simulink model "Heading_Guide_110"  (Simulink 8.7)
settings: Solver=ode45  StartTime=0.0  StopTime=10.0  RelTol=1e-3
undefined symbols (not defined in the file or in its folder): DiscIntNeverNeededParam
libraries: simulink x1, discretizing x1
settings Model: Creator=arnaud  LastModifiedBy=bourbouh
settings DataIOCC: SignalLoggingSaveFormat=ModelDataLogs
settings OptimizationCC: ExpressionDepthLimit=2147483647
settings DebuggingCC: SolverPrmCheckMsg=warning  FcnCallInpInsideContextMsg=UseLocalSettings  StateNameClashWarn=warning  StrictBusMsg=Warning
settings GRTTargetCC: GeneratePreprocessorConditionals=Use local settings  CombineOutputUpdateFcns=off  GRTInterface=on

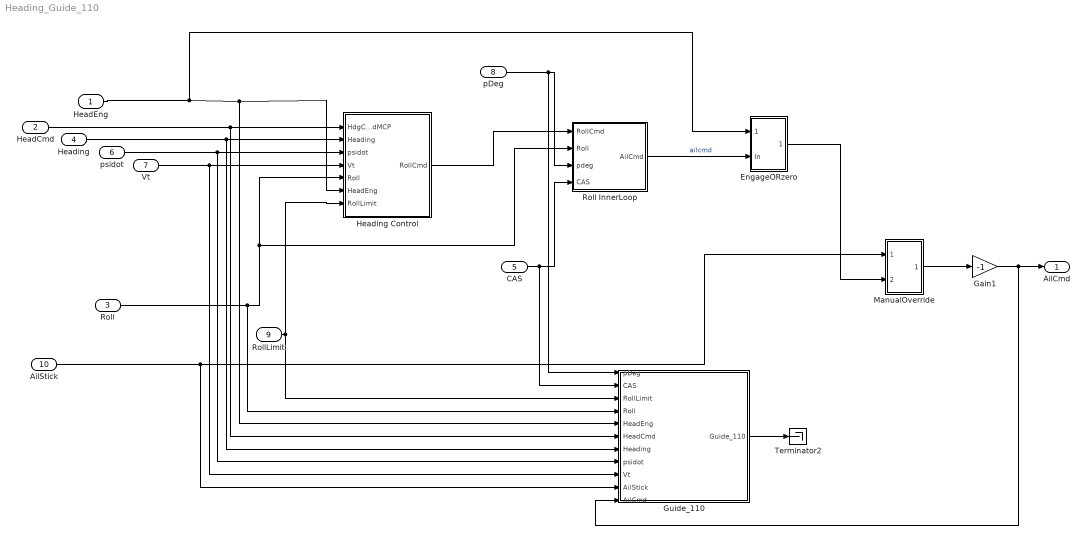
== system Heading_Guide_110 ==
  HeadEng : Inport  OutDataTypeStr=boolean
  HeadCmd : Inport  Port=2  OutDataTypeStr=double
  Roll : Inport  Port=3  OutDataTypeStr=double
  Heading : Inport  Port=4  OutDataTypeStr=double
  CAS : Inport  Port=5  OutDataTypeStr=double
  psidot : Inport  Port=6  OutDataTypeStr=double
  Vt : Inport  Port=7  OutDataTypeStr=double
  pDeg : Inport  Port=8  OutDataTypeStr=double
  RollLimit : Inport  Port=9  OutDataTypeStr=double
  AilStick : Inport  Port=10  OutDataTypeStr=double
  EngageORzero : Subsystem
  Gain1 : Gain  RequirementInfo={} %GIDa_2f421c02_996e_46c9_ac2a_3c25b016b229  Gain=-1  SaturateOnIntegerOverflow=on  OutDataTypeStr=Inherit: Same as input  ParamDataTypeStr=Inherit: Same as input
  Guide_110 : Subsystem  TreatAsAtomicUnit=on  mask(Observer){AnnotationType=ensures, ObserverType=ellipsoid}
      mask prompts: AnnotationType "Type of annotation (pre/post...)"; ObserverType "Observer type"
      mask help:
      | Set an observer for the system.
      | The annotation type parameter sets the type of observer:
      | - requires : pre-condition
      | - ensures : post-condition
      | - assert : an assertion
      | - observer : the observer computes a special type of properties
      mask TypeOptions AnnotationType: ensures | requires | assert | observer
      mask Callback AnnotationType:
      | paramStr = get_param(gcb, 'MaskValues');
      | 
      | if strcmp(paramStr{1}(1),'o')
      |     set_param(gcb,'MaskVisibilities',{'on';'on'});
      |     paramStr{2} = 'ellipsoid';
      |     set_param(gcb,'MaskValues',paramStr);
      | else
      |     set_param(gcb,'MaskVisibilities',{'on';'off'});
      | end
      mask Callback ObserverType:
      | paramStr = get_param(gcb, 'MaskValues');
      | 
      | if strcmp(paramStr{1}(1),'observer')
      |     set_param(gcb,'MaskVisibilities',{'on';'on'});
      |     paramStr{2} = 'ellipsoid';
      |     set_param(gcb,'MaskValues',paramStr);
      | else
      |     set_param(gcb,'MaskVisibilities',{'on';'off'});
      | end
      mask Display:
      | color('red');
      | text(0.5, 0.5, 'Observer Block', 'horizontalAlignment', 'center');
  Heading Control : Subsystem  RequirementInfo={'other' '..\..\tcm_requirements.docx' '@Simulink_requirement_item_16' 'true' 'Heading Control' '' }  TreatAsAtomicUnit=on
  ManualOverride : Subsystem
  Roll InnerLoop : Subsystem  RequirementInfo={'other' '..\..\tcm_requirements.docx' '@Simulink_requirement_item_18' 'true' 'Roll InnerLoop' '' }  TreatAsAtomicUnit=on
  Terminator2 : Terminator
  AilCmd : Outport
  wires:
  pDeg/1 -> Roll InnerLoop/3(pdeg), Guide_110/1(pDeg)
  Vt/1 -> Heading Control/4(Vt), Guide_110/9(Vt)
  psidot/1 -> Heading Control/3(psidot), Guide_110/8(psidot)
  Heading/1 -> Heading Control/2(Heading), Guide_110/7(Heading)
  Roll/1 -> Heading Control/5(Roll), Roll InnerLoop/2(Roll), Guide_110/4(Roll)
  Heading Control/1(RollCmd) -> Roll InnerLoop/1(RollCmd)
  Roll InnerLoop/1(AilCmd) -> EngageORzero/2(In)  "ailcmd"
  HeadEng/1 -> EngageORzero/1(Engage), Heading Control/6(HeadEng), Guide_110/5(HeadEng)
  CAS/1 -> Roll InnerLoop/4(CAS), Guide_110/2(CAS)
  RollLimit/1 -> Heading Control/7(RollLimit), Guide_110/3(RollLimit)
  ManualOverride/1(Out) -> Gain1/1
  AilStick/1 -> ManualOverride/1(Man), Guide_110/10(AilStick)
  Gain1/1 -> AilCmd/1, Guide_110/11(AilCmd)
  EngageORzero/1(Out) -> ManualOverride/2(Auto)
  HeadCmd/1 -> Heading Control/1(HdgCmdMCP), Guide_110/6(HeadCmd)
  Guide_110/1(Guide_110) -> Terminator2/1

== system Heading_Guide_110/EngageORzero ==
  Engage : Inport
  In : Inport  Port=2
  Logical Operator5 : Logic  RequirementInfo={} %GIDa_7add67f6_200e_4459_8afc_a50a3802c341  AllPortsSameDT=off  OutDataTypeStr=boolean
  Switch1 : Switch  RequirementInfo={} %GIDa_a1777089_6daf_41d2_9e69_9356c4782e25  Threshold=0.5
  zero10 : Constant  RequirementInfo={} %GIDa_d889400f_b153_4cfc_a180_15b84145f1e0
  zero9 : Constant  RequirementInfo={} %GIDa_9027fd24_3b48_4acd_a774_517fb1aa3516  Value=0
  Out : Outport
  wires:
  Engage/1 -> Logical Operator5/1
  zero10/1 -> Logical Operator5/2
  zero9/1 -> Switch1/3
  In/1 -> Switch1/1
  Logical Operator5/1 -> Switch1/2
  Switch1/1 -> Out/1

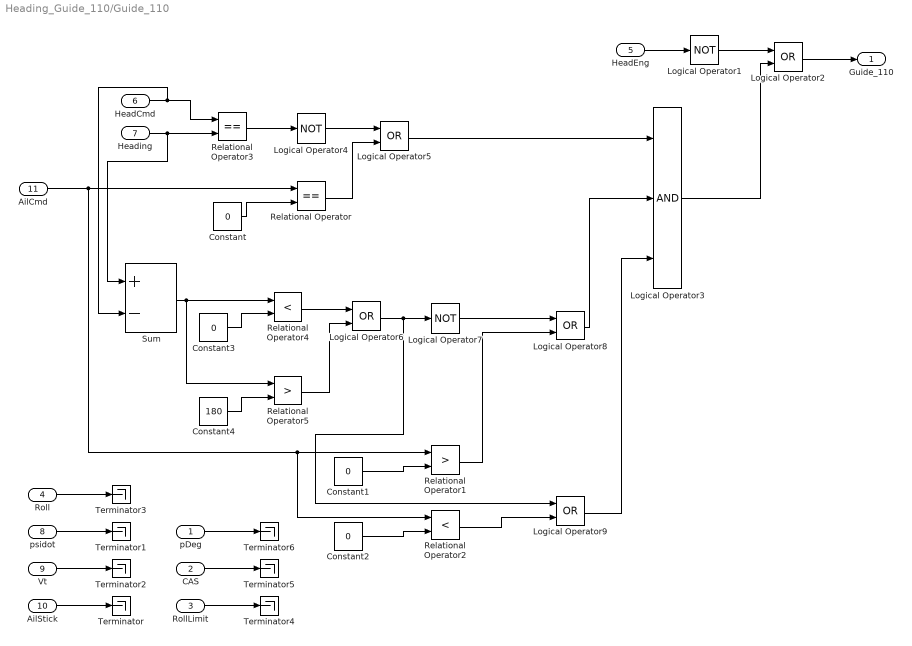
== system Heading_Guide_110/Guide_110 ==
  pDeg : Inport
  CAS : Inport  Port=2
  RollLimit : Inport  Port=3
  Roll : Inport  Port=4
  HeadEng : Inport  Port=5
  HeadCmd : Inport  Port=6
  Heading : Inport  Port=7
  psidot : Inport  Port=8
  Vt : Inport  Port=9
  AilStick : Inport  Port=10
  AilCmd : Inport  Port=11
  Constant{,1..3} (4 alike) : Constant  Value=0
  Constant4 : Constant  Value=180
  Logical Operator1 : Logic  Operator=NOT  AllPortsSameDT=off  OutDataTypeStr=boolean
  Logical Operator{2,5..6,8..9} (5 alike) : Logic  Operator=OR  AllPortsSameDT=off  OutDataTypeStr=boolean
  Logical Operator3 : Logic  Inputs=3  AllPortsSameDT=off  OutDataTypeStr=boolean
  Logical Operator4 : Logic  Operator=NOT  AllPortsSameDT=off  OutDataTypeStr=boolean
  Logical Operator7 : Logic  Operator=NOT  AllPortsSameDT=off  OutDataTypeStr=boolean
  Relational Operator : RelationalOperator  Operator===  OutDataTypeStr=boolean
  Relational Operator1 : RelationalOperator  Operator=>  OutDataTypeStr=boolean
  Relational Operator2 : RelationalOperator  Operator=<  OutDataTypeStr=boolean
  Relational Operator3 : RelationalOperator  Operator===  OutDataTypeStr=boolean
  Relational Operator4 : RelationalOperator  Operator=<  OutDataTypeStr=boolean
  Relational Operator5 : RelationalOperator  Operator=>  OutDataTypeStr=boolean
  Sum : Sum  Inputs=+-
  Terminator{,1..6} (7 alike) : Terminator
  Guide_110 : Outport
  wires:
  AilStick/1 -> Terminator/1
  Vt/1 -> Terminator2/1
  psidot/1 -> Terminator1/1
  Roll/1 -> Terminator3/1
  RollLimit/1 -> Terminator4/1
  CAS/1 -> Terminator5/1
  pDeg/1 -> Terminator6/1
  HeadEng/1 -> Logical Operator1/1
  Logical Operator1/1 -> Logical Operator2/1
  Logical Operator2/1 -> Guide_110/1
  AilCmd/1 -> Relational Operator/1, Relational Operator1/1, Relational Operator2/1
  Constant/1 -> Relational Operator/2
  Constant1/1 -> Relational Operator1/2
  Constant2/1 -> Relational Operator2/2
  Logical Operator4/1 -> Logical Operator5/1
  Relational Operator3/1 -> Logical Operator4/1
  Relational Operator/1 -> Logical Operator5/2
  Logical Operator5/1 -> Logical Operator3/1
  Sum/1 -> Relational Operator4/1, Relational Operator5/1
  Constant3/1 -> Relational Operator4/2
  Relational Operator4/1 -> Logical Operator6/1
  Constant4/1 -> Relational Operator5/2
  Relational Operator5/1 -> Logical Operator6/2
  HeadCmd/1 -> Relational Operator3/1, Sum/2
  Heading/1 -> Relational Operator3/2, Sum/1
  Logical Operator6/1 -> Logical Operator7/1, Logical Operator9/1
  Logical Operator7/1 -> Logical Operator8/1
  Relational Operator1/1 -> Logical Operator8/2
  Logical Operator8/1 -> Logical Operator3/2
  Relational Operator2/1 -> Logical Operator9/2
  Logical Operator9/1 -> Logical Operator3/3
  Logical Operator3/1 -> Logical Operator2/2

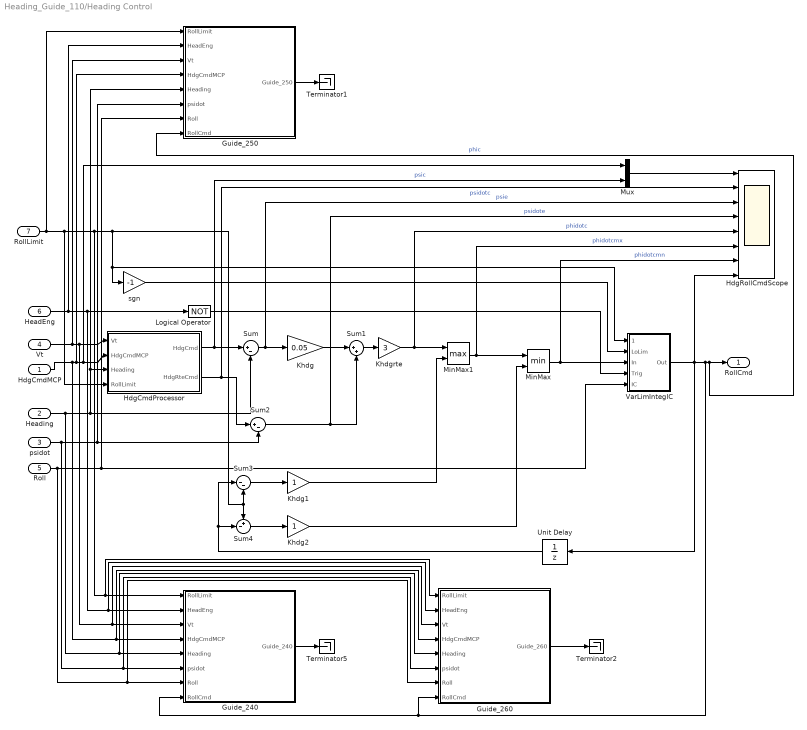
== system Heading_Guide_110/Heading Control ==
  HdgCmdMCP : Inport  RequirementInfo={} %GIDa_afcd05d1_a9dc_45a7_a8f8_7136ccc61726
  Heading : Inport  RequirementInfo={} %GIDa_19b80fe4_d265_482c_b709_18db80a7cdf3  Port=2
  psidot : Inport  RequirementInfo={} %GIDa_e421e82d_0cc7_4ad7_ac7a_9fb430d189d5  Port=3
  Vt : Inport  RequirementInfo={} %GIDa_9daf3e20_e00e_4f36_b534_d9747a241338  Port=4
  Roll : Inport  RequirementInfo={} %GIDa_8629ba77_a751_4097_af53_617eaa1017be  Port=5
  HeadEng : Inport  RequirementInfo={} %GIDa_dadb1310_2bf4_48cf_8970_85174d784ee3  Port=6
  RollLimit : Inport  Port=7
  Guide_240 : Subsystem  TreatAsAtomicUnit=on  mask(Observer){AnnotationType=ensures, ObserverType=ellipsoid}
      mask prompts: AnnotationType "Type of annotation (pre/post...)"; ObserverType "Observer type"
      mask help:
      | Set an observer for the system.
      | The annotation type parameter sets the type of observer:
      | - requires : pre-condition
      | - ensures : post-condition
      | - assert : an assertion
      | - observer : the observer computes a special type of properties
      mask TypeOptions AnnotationType: ensures | requires | assert | observer
      mask Callback AnnotationType:
      | paramStr = get_param(gcb, 'MaskValues');
      | 
      | if strcmp(paramStr{1}(1),'o')
      |     set_param(gcb,'MaskVisibilities',{'on';'on'});
      |     paramStr{2} = 'ellipsoid';
      |     set_param(gcb,'MaskValues',paramStr);
      | else
      |     set_param(gcb,'MaskVisibilities',{'on';'off'});
      | end
      mask Callback ObserverType:
      | paramStr = get_param(gcb, 'MaskValues');
      | 
      | if strcmp(paramStr{1}(1),'observer')
      |     set_param(gcb,'MaskVisibilities',{'on';'on'});
      |     paramStr{2} = 'ellipsoid';
      |     set_param(gcb,'MaskValues',paramStr);
      | else
      |     set_param(gcb,'MaskVisibilities',{'on';'off'});
      | end
      mask Display:
      | color('red');
      | text(0.5, 0.5, 'Observer Block', 'horizontalAlignment', 'center');
  Guide_250 : Subsystem  TreatAsAtomicUnit=on  mask(Observer){AnnotationType=ensures, ObserverType=ellipsoid}
      mask prompts: AnnotationType "Type of annotation (pre/post...)"; ObserverType "Observer type"
      mask help:
      | Set an observer for the system.
      | The annotation type parameter sets the type of observer:
      | - requires : pre-condition
      | - ensures : post-condition
      | - assert : an assertion
      | - observer : the observer computes a special type of properties
      mask TypeOptions AnnotationType: ensures | requires | assert | observer
      mask Callback AnnotationType:
      | paramStr = get_param(gcb, 'MaskValues');
      | 
      | if strcmp(paramStr{1}(1),'o')
      |     set_param(gcb,'MaskVisibilities',{'on';'on'});
      |     paramStr{2} = 'ellipsoid';
      |     set_param(gcb,'MaskValues',paramStr);
      | else
      |     set_param(gcb,'MaskVisibilities',{'on';'off'});
      | end
      mask Callback ObserverType:
      | paramStr = get_param(gcb, 'MaskValues');
      | 
      | if strcmp(paramStr{1}(1),'observer')
      |     set_param(gcb,'MaskVisibilities',{'on';'on'});
      |     paramStr{2} = 'ellipsoid';
      |     set_param(gcb,'MaskValues',paramStr);
      | else
      |     set_param(gcb,'MaskVisibilities',{'on';'off'});
      | end
      mask Display:
      | color('red');
      | text(0.5, 0.5, 'Observer Block', 'horizontalAlignment', 'center');
  Guide_260 : Subsystem  TreatAsAtomicUnit=on  mask(Observer){AnnotationType=ensures, ObserverType=ellipsoid}
      mask prompts: AnnotationType "Type of annotation (pre/post...)"; ObserverType "Observer type"
      mask help:
      | Set an observer for the system.
      | The annotation type parameter sets the type of observer:
      | - requires : pre-condition
      | - ensures : post-condition
      | - assert : an assertion
      | - observer : the observer computes a special type of properties
      mask TypeOptions AnnotationType: ensures | requires | assert | observer
      mask Callback AnnotationType:
      | paramStr = get_param(gcb, 'MaskValues');
      | 
      | if strcmp(paramStr{1}(1),'o')
      |     set_param(gcb,'MaskVisibilities',{'on';'on'});
      |     paramStr{2} = 'ellipsoid';
      |     set_param(gcb,'MaskValues',paramStr);
      | else
      |     set_param(gcb,'MaskVisibilities',{'on';'off'});
      | end
      mask Callback ObserverType:
      | paramStr = get_param(gcb, 'MaskValues');
      | 
      | if strcmp(paramStr{1}(1),'observer')
      |     set_param(gcb,'MaskVisibilities',{'on';'on'});
      |     paramStr{2} = 'ellipsoid';
      |     set_param(gcb,'MaskValues',paramStr);
      | else
      |     set_param(gcb,'MaskVisibilities',{'on';'off'});
      | end
      mask Display:
      | color('red');
      | text(0.5, 0.5, 'Observer Block', 'horizontalAlignment', 'center');
  HdgCmdProcessor : Subsystem  RequirementInfo={} %GIDa_3cb77e5f_f630_4f22_88a8_7528bfceb83f
  HdgRollCmdScope : Scope  NumInputPorts=8
      settings: RequirementInfo={} %GIDa_5fbe2135_fdf1_4f64_a179_faa1710ae21e
  Khdg : Gain  RequirementInfo={} %GIDa_abf81b08_c210_4343_b4da_5a7e229caeb6  Gain=0.05
  Khdg1 : Gain  RequirementInfo={} %GIDa_7a7a35ca_24a5_4d20_bc30_55deea16462c
  Khdg2 : Gain  RequirementInfo={} %GIDa_57191899_7ee5_4454_897a_7009651ed5fb
  Khdgrte : Gain  RequirementInfo={} %GIDa_bcc6a420_18f3_43f0_aaa1_aaa1bbf90f64  Gain=3
  Logical Operator : Logic  RequirementInfo={} %GIDa_5ad405ac_0a88_4b96_aa0e_75483351ee25  Operator=NOT  AllPortsSameDT=off  OutDataTypeStr=boolean
  MinMax : MinMax  RequirementInfo={} %GIDa_4b9381d8_eb85_418b_a975_85846d5ca8c2  Inputs=2
  MinMax1 : MinMax  RequirementInfo={} %GIDa_b40e082d_0fb2_4088_baf4_e9a71be9bcc1  Function=max  Inputs=2
  Mux : Mux  RequirementInfo={} %GIDa_0e83f6c6_ae04_43dd_95fe_a79ec32b40e2  Inputs=2
  Sum : Sum  RequirementInfo={} %GIDa_b89885fc_f86c_4a50_8ce5_47d0488bdc1c  Inputs=|+-
  Sum1 : Sum  RequirementInfo={} %GIDa_40ec6862_b1f8_4f97_ae14_1eadabbceb30  Inputs=|++
  Sum2 : Sum  RequirementInfo={} %GIDa_307d6880_3ab8_4deb_90e0_d68f11d87c85  Inputs=|+-
  Sum3 : Sum  RequirementInfo={} %GIDa_ebb8b765_7f4a_435f_be61_680d3199141b  Inputs=|--
  Sum4 : Sum  RequirementInfo={} %GIDa_05638559_562a_476e_9e4c_91124434a43b  Inputs=+-|
  Terminator1 : Terminator
  Terminator2 : Terminator
  Terminator5 : Terminator
  Unit Delay : UnitDelay  SampleTime=-1
  VarLimIntegIC : Subsystem  RequirementInfo={} %GIDa_7da7eaf5_9731_498e_9aad_b41279918004
  sgn : Gain  RequirementInfo={} %GIDa_84e2dc00_f2e5_41f4_89ce_c9fef234974f  Gain=-1
  RollCmd : Outport  RequirementInfo={} %GIDa_aa862f7f_5d4e_408f_b8c4_26b4ce96fbda
  wires:
  Heading/1 -> Guide_250/5(Heading), HdgCmdProcessor/3(Heading), Sum/2, Guide_240/5(Heading), Guide_260/5(Heading)
  HdgCmdProcessor/1(HdgCmd) -> Sum/1, Mux/2  "psic"
  Sum/1 -> Khdg/1, HdgRollCmdScope/3  "psie"
  Khdg/1 -> Sum1/1
  Sum2/1 -> Sum1/2, HdgRollCmdScope/4  "psidote"
  HdgCmdProcessor/2(HdgRteCmd) -> Sum2/1, HdgRollCmdScope/2  "psidotc"
  psidot/1 -> Sum2/2, Guide_250/6(psidot), Guide_240/6(psidot), Guide_260/6(psidot)
  Vt/1 -> HdgCmdProcessor/1(Vt), Guide_240/3(Vt), Guide_260/3(Vt), Guide_250/3(Vt)
  HdgCmdMCP/1 -> HdgCmdProcessor/2(HdgCmdMCP), Mux/1, Guide_250/4(HdgCmdMCP), Guide_240/4(HdgCmdMCP), Guide_260/4(HdgCmdMCP)
  VarLimIntegIC/1(Out) -> Unit Delay/1, HdgRollCmdScope/8, RollCmd/1, Guide_250/8(RollCmd), Guide_240/8(RollCmd), Guide_260/8(RollCmd)  "phic"
  RollLimit/1 -> Sum4/1, Sum3/2, VarLimIntegIC/1(UpLim), sgn/1, Guide_240/1(RollLimit), Guide_260/1(RollLimit), HdgCmdProcessor/4(RollLimit), Guide_250/1(RollLimit)
  sgn/1 -> VarLimIntegIC/2(LoLim)
  Sum1/1 -> Khdgrte/1
  MinMax1/1 -> MinMax/1, HdgRollCmdScope/6  "phidotcmx"
  MinMax/1 -> VarLimIntegIC/3(In), HdgRollCmdScope/7  "phidotcmn"
  HeadEng/1 -> Logical Operator/1, Guide_240/2(HeadEng), Guide_260/2(HeadEng), Guide_250/2(HeadEng)
  Sum3/1 -> Khdg1/1
  Sum4/1 -> Khdg2/1
  Khdg1/1 -> MinMax1/2
  Khdg2/1 -> MinMax/2
  Roll/1 -> VarLimIntegIC/5(IC), Guide_250/7(Roll), Guide_240/7(Roll), Guide_260/7(Roll)
  Khdgrte/1 -> MinMax1/1, HdgRollCmdScope/5  "phidotc"
  Logical Operator/1 -> VarLimIntegIC/4(Trig)
  Mux/1 -> HdgRollCmdScope/1
  Guide_240/1(Guide_240) -> Terminator5/1
  Guide_250/1(Guide_250) -> Terminator1/1
  Guide_260/1(Guide_260) -> Terminator2/1
  Unit Delay/1 -> Sum3/1, Sum4/2

== system Heading_Guide_110/ManualOverride ==
  Man : Inport
  Auto : Inport  Port=2
  Switch1 : Switch  RequirementInfo={} %GIDa_5800ea93_45af_42da_974c_4cd975d0b8c8  Criteria=u2 ~= 0  Threshold=0.5
  Out : Outport
  wires:
  Man/1 -> Switch1/3, Switch1/2
  Auto/1 -> Switch1/1
  Switch1/1 -> Out/1

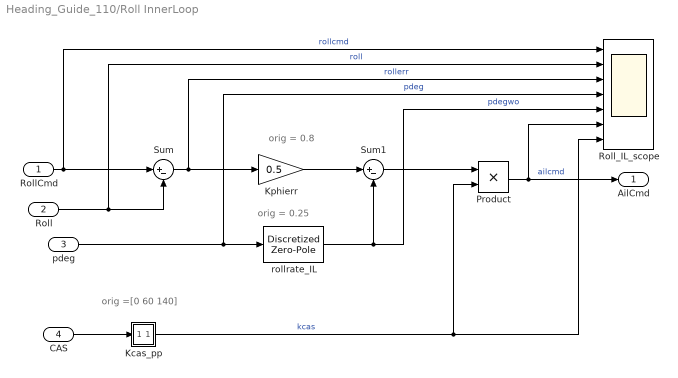
== system Heading_Guide_110/Roll InnerLoop ==
  note: orig =[0 60 140]
  note: orig = 0.25
  note: orig = 0.8
  RollCmd : Inport  RequirementInfo={} %GIDa_549f9d91_ca5c_4ec7_bf56_cf05f3793396
  Roll : Inport  RequirementInfo={} %GIDa_d885705c_af8c_4e18_b4d1_2f073687ea2c  Port=2
  pdeg : Inport  RequirementInfo={} %GIDa_ba7aa095_15b8_4f85_9051_8b947d28a24d  Port=3
  CAS : Inport  RequirementInfo={} %GIDa_defe4f55_1722_479a_b684_dc07a497c4ef  Port=4
  Kcas_pp : Subsystem  TreatAsAtomicUnit=on
  Kphierr : Gain  RequirementInfo={} %GIDa_96c602a9_a07d_4519_9a2c_04c20a8c958d  Gain=0.5
  Product : Product  RequirementInfo={} %GIDa_6029a1e1_bbec_4e58_a2a6_3f9df62d6e90  RndMeth=Zero
  Roll_IL_scope : Scope  NumInputPorts=7
      settings: RequirementInfo={} %GIDa_ec5ee575_c049_4397_a5dd_5347629f97a6
  Sum : Sum  RequirementInfo={} %GIDa_6dd565f9_cc9c_463a_985b_c182e040d7fd  Inputs=|+-
  Sum1 : Sum  RequirementInfo={} %GIDa_02561aa6_0360_4e6c_b76e_5dde7f2ab3b1  Inputs=|+-
  rollrate_IL : discretizing/Discretized Zero-Pole  RequirementInfo={} %GIDa_636569be_bc7e_4244_84a4_4a62b7fc0808  SystemSampleTime=-1  Zeros=0  Poles=-0.5  Gain=0.00645  AbsTol=auto  SampleTime=1.0  method=zoh  Wc=1
  AilCmd : Outport  RequirementInfo={} %GIDa_cd7ddcd8_c7c7_43e2_be4e_2c0bb3f4c702
  wires:
  Product/1 -> AilCmd/1, Roll_IL_scope/6  "ailcmd"
  Kcas_pp/1(Out) -> Product/2, Roll_IL_scope/7  "kcas"
  Sum1/1 -> Product/1
  CAS/1 -> Kcas_pp/1(In)
  rollrate_IL/1 -> Sum1/2, Roll_IL_scope/5  "pdegwo"
  pdeg/1 -> rollrate_IL/1, Roll_IL_scope/4  "pdeg"
  Kphierr/1 -> Sum1/1
  Roll/1 -> Sum/2, Roll_IL_scope/2  "roll"
  Sum/1 -> Kphierr/1, Roll_IL_scope/3  "rollerr"
  RollCmd/1 -> Sum/1, Roll_IL_scope/1  "rollcmd"

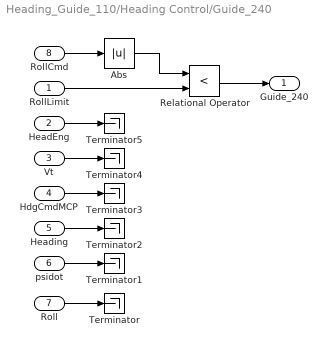
== system Heading_Guide_110/Heading Control/Guide_240 ==
  RollLimit : Inport
  HeadEng : Inport  Port=2
  Vt : Inport  Port=3
  HdgCmdMCP : Inport  Port=4
  Heading : Inport  Port=5
  psidot : Inport  Port=6
  Roll : Inport  Port=7
  RollCmd : Inport  Port=8
  Abs : Abs
  Relational Operator : RelationalOperator  Operator=<  OutDataTypeStr=boolean
  Terminator{,1..5} (6 alike) : Terminator
  Guide_240 : Outport
  wires:
  Roll/1 -> Terminator/1
  HeadEng/1 -> Terminator5/1
  Vt/1 -> Terminator4/1
  HdgCmdMCP/1 -> Terminator3/1
  Heading/1 -> Terminator2/1
  psidot/1 -> Terminator1/1
  RollCmd/1 -> Abs/1
  Abs/1 -> Relational Operator/1
  RollLimit/1 -> Relational Operator/2
  Relational Operator/1 -> Guide_240/1

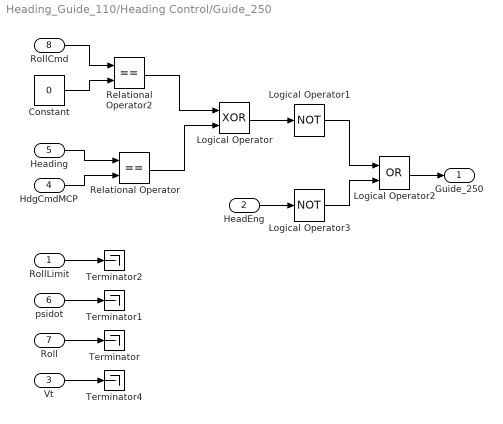
== system Heading_Guide_110/Heading Control/Guide_250 ==
  RollLimit : Inport
  HeadEng : Inport  Port=2
  Vt : Inport  Port=3
  HdgCmdMCP : Inport  Port=4
  Heading : Inport  Port=5
  psidot : Inport  Port=6
  Roll : Inport  Port=7
  RollCmd : Inport  Port=8
  Constant : Constant  Value=0
  Logical Operator : Logic  Operator=XOR  AllPortsSameDT=off  OutDataTypeStr=boolean
  Logical Operator1 : Logic  Operator=NOT  AllPortsSameDT=off  OutDataTypeStr=boolean
  Logical Operator2 : Logic  Operator=OR  AllPortsSameDT=off  OutDataTypeStr=boolean
  Logical Operator3 : Logic  Operator=NOT  AllPortsSameDT=off  OutDataTypeStr=boolean
  Relational Operator : RelationalOperator  Operator===  OutDataTypeStr=boolean
  Relational Operator2 : RelationalOperator  Operator===  OutDataTypeStr=boolean
  Terminator{,1..2,4} (4 alike) : Terminator
  Guide_250 : Outport
  wires:
  Roll/1 -> Terminator/1
  Vt/1 -> Terminator4/1
  psidot/1 -> Terminator1/1
  RollLimit/1 -> Terminator2/1
  Heading/1 -> Relational Operator/1
  HdgCmdMCP/1 -> Relational Operator/2
  RollCmd/1 -> Relational Operator2/1
  Constant/1 -> Relational Operator2/2
  Relational Operator2/1 -> Logical Operator/1
  Relational Operator/1 -> Logical Operator/2
  Logical Operator/1 -> Logical Operator1/1
  HeadEng/1 -> Logical Operator3/1
  Logical Operator1/1 -> Logical Operator2/1
  Logical Operator3/1 -> Logical Operator2/2
  Logical Operator2/1 -> Guide_250/1

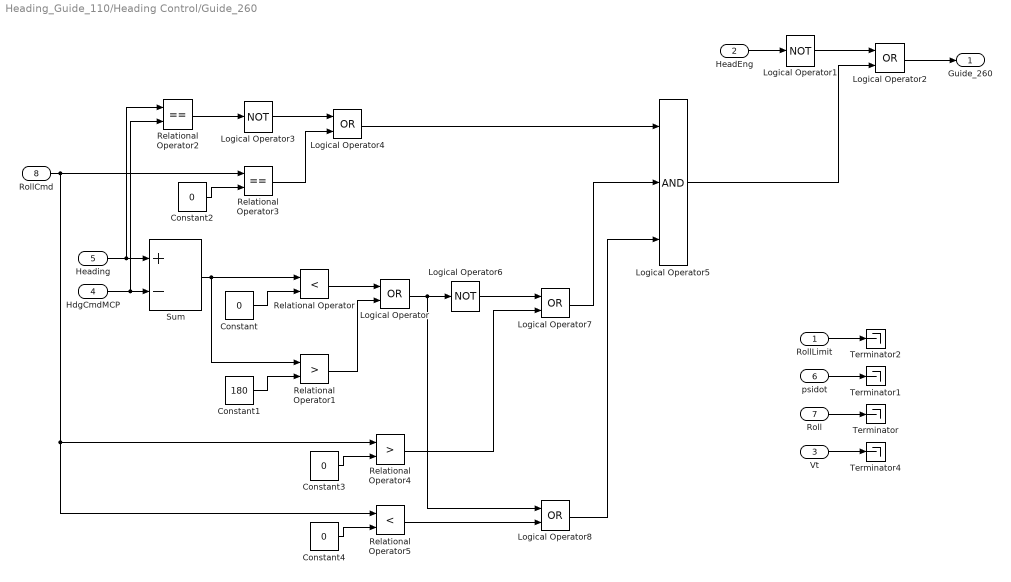
== system Heading_Guide_110/Heading Control/Guide_260 ==
  RollLimit : Inport
  HeadEng : Inport  Port=2
  Vt : Inport  Port=3
  HdgCmdMCP : Inport  Port=4
  Heading : Inport  Port=5
  psidot : Inport  Port=6
  Roll : Inport  Port=7
  RollCmd : Inport  Port=8
  Constant{,2..4} (4 alike) : Constant  Value=0
  Constant1 : Constant  Value=180
  Logical Operator{,2,4,7..8} (5 alike) : Logic  Operator=OR  AllPortsSameDT=off  OutDataTypeStr=boolean
  Logical Operator1 : Logic  Operator=NOT  AllPortsSameDT=off  OutDataTypeStr=boolean
  Logical Operator3 : Logic  Operator=NOT  AllPortsSameDT=off  OutDataTypeStr=boolean
  Logical Operator5 : Logic  Inputs=3  AllPortsSameDT=off  OutDataTypeStr=boolean
  Logical Operator6 : Logic  Operator=NOT  AllPortsSameDT=off  OutDataTypeStr=boolean
  Relational Operator : RelationalOperator  Operator=<  OutDataTypeStr=boolean
  Relational Operator1 : RelationalOperator  Operator=>  OutDataTypeStr=boolean
  Relational Operator2 : RelationalOperator  Operator===  OutDataTypeStr=boolean
  Relational Operator3 : RelationalOperator  Operator===  OutDataTypeStr=boolean
  Relational Operator4 : RelationalOperator  Operator=>  OutDataTypeStr=boolean
  Relational Operator5 : RelationalOperator  Operator=<  OutDataTypeStr=boolean
  Sum : Sum  Inputs=+-
  Terminator{,1..2,4} (4 alike) : Terminator
  Guide_260 : Outport
  wires:
  Roll/1 -> Terminator/1
  Vt/1 -> Terminator4/1
  psidot/1 -> Terminator1/1
  RollLimit/1 -> Terminator2/1
  Heading/1 -> Sum/1, Relational Operator2/1
  HdgCmdMCP/1 -> Sum/2, Relational Operator2/2
  Sum/1 -> Relational Operator/1, Relational Operator1/1
  Constant/1 -> Relational Operator/2
  Relational Operator/1 -> Logical Operator/1
  Constant1/1 -> Relational Operator1/2
  Relational Operator1/1 -> Logical Operator/2
  HeadEng/1 -> Logical Operator1/1
  Logical Operator1/1 -> Logical Operator2/1
  Logical Operator2/1 -> Guide_260/1
  Logical Operator3/1 -> Logical Operator4/1
  Relational Operator2/1 -> Logical Operator3/1
  RollCmd/1 -> Relational Operator3/1, Relational Operator4/1, Relational Operator5/1
  Constant2/1 -> Relational Operator3/2
  Relational Operator3/1 -> Logical Operator4/2
  Logical Operator4/1 -> Logical Operator5/1
  Constant3/1 -> Relational Operator4/2
  Logical Operator/1 -> Logical Operator6/1, Logical Operator8/1
  Logical Operator6/1 -> Logical Operator7/1
  Relational Operator4/1 -> Logical Operator7/2
  Logical Operator7/1 -> Logical Operator5/2
  Constant4/1 -> Relational Operator5/2
  Relational Operator5/1 -> Logical Operator8/2
  Logical Operator8/1 -> Logical Operator5/3
  Logical Operator5/1 -> Logical Operator2/2

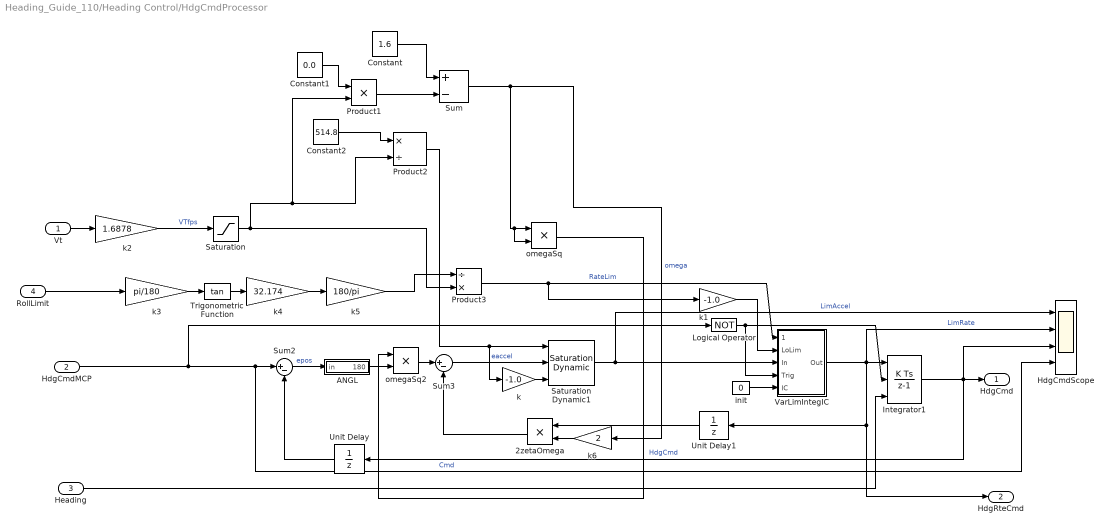
== system Heading_Guide_110/Heading Control/HdgCmdProcessor ==
  Vt : Inport  RequirementInfo={} %GIDa_aea371ad_7692_43c3_9333_237397a7088d
  HdgCmdMCP : Inport  RequirementInfo={} %GIDa_62146feb_aace_4fc2_8116_9e6cd7e3722f  Port=2
  Heading : Inport  RequirementInfo={} %GIDa_2367d888_2282_4a9b_9dc0_ce749bdb20fa  Port=3
  RollLimit : Inport  Port=4
  2zetaOmega : Product  RequirementInfo={} %GIDa_f321de1d_2313_4525_97dc_b8d5cf0673a7  RndMeth=Zero
  ANGL : Subsystem  RequirementInfo={} %GIDa_a65114d8_8cfa_43a6_b93e_efba84d5b466
  Constant : Constant  Value=1.6
  Constant1 : Constant  Value=0.0
  Constant2 : Constant  Value=514.8
  HdgCmdScope : Scope  NumInputPorts=4
      settings: RequirementInfo={} %GIDa_44f9dfb2_1047_4c85_9993_6df91b14ae0d
  Integrator1 : DiscreteIntegrator  ExternalReset=level  InitialConditionSource=external  SampleTime=1.0  ICPrevOutput=DiscIntNeverNeededParam  ICPrevScaledInput=DiscIntNeverNeededParam  mask(DiscretizedDiscreteIntegrator){}
      mask init:
      | %zoh
  Logical Operator : Logic  RequirementInfo={} %GIDa_a3be1b8e_7e30_4ddb_8576_d6096a49c77e  Operator=NOT  AllPortsSameDT=off  OutDataTypeStr=boolean
  Product1 : Product  RndMeth=Zero
  Product2 : Product  Inputs=*/  RndMeth=Zero
  Product3 : Product  Inputs=/*  RndMeth=Zero
  Saturation : Saturate  RequirementInfo={} %GIDa_34361c95_77fe_4878_a89a_f2e2245d083f  UpperLimit=1000  LowerLimit=0.0001
  Saturation Dynamic1 : simulink/Discontinuities/Saturation Dynamic  RequirementInfo={} %GIDa_3c1bb0e4_035b_467b_b908_73d0679fa8c4  OutMin=[]  OutMax=[]  OutDataTypeStr=Inherit: Same as second input  OutDataType=fixdt(1, 16)  OutScaling=2^-10  DoSatur=off
  Sum : Sum  Inputs=+-
  Sum2 : Sum  RequirementInfo={} %GIDa_0134b7ed_8c9c_449a_ac58_c6bc449e5dc3  Inputs=|+-
  Sum3 : Sum  RequirementInfo={} %GIDa_133a47a4_a1d1_45cf_bb65_a8e707312c61  Inputs=|+-
  Trigonometric Function : Trigonometry  RequirementInfo={} %GIDa_9fedb248_844e_457e_a851_4a39016fb810  Operator=tan
  Unit Delay : UnitDelay  SampleTime=-1
  Unit Delay1 : UnitDelay  SampleTime=-1
  VarLimIntegIC : Subsystem  RequirementInfo={} %GIDa_5e236912_7c4b_441a_a6c7_d31391da156a
  init : Constant  RequirementInfo={} %GIDa_bb6a6882_f5a4_4f54_8f02_3d74a10327cc  Value=0
  k : Gain  RequirementInfo={} %GIDa_b3adcecb_db12_4f0e_a73c_fd191106ac98  Gain=-1.0
  k1 : Gain  RequirementInfo={} %GIDa_4080639b_e5dd_4b50_81e0_40e346cb6275  Gain=-1.0
  k2 : Gain  RequirementInfo={} %GIDa_3129ff2a_7a94_46f5_a52d_bf604afbaa9d  Gain=1.6878
  k3 : Gain  RequirementInfo={} %GIDa_bc42355c_264a_47e1_8506_c4c4e8e068fc  Gain=pi/180
  k4 : Gain  RequirementInfo={} %GIDa_0e3e2a32_c8b7_428f_ab0c_0faebbbf5e76  Gain=32.174
  k5 : Gain  RequirementInfo={} %GIDa_be5380e6_e279_4fba_b4a2_cea2808c46f4  Gain=180/pi
  k6 : Gain  RequirementInfo={} %GIDa_bccc5425_7281_49cf_93c6_a752e7732049  Gain=2
  omegaSq : Product  RequirementInfo={} %GIDa_e5c95743_58d1_4d7b_8e0f_0d5dca474f7a  RndMeth=Zero
  omegaSq2 : Product  RequirementInfo={} %GIDa_907b30dd_aede_4316_9a8a_044ea704cef8  RndMeth=Zero
  HdgCmd : Outport  RequirementInfo={} %GIDa_7c7f0b37_435d_4e7c_952c_62c879fcb657
  HdgRteCmd : Outport  RequirementInfo={} %GIDa_0b79bbaa_a2da_4cb9_814f_266c555013e7  Port=2
  wires:
  Integrator1/1 -> Unit Delay/1, HdgCmd/1, HdgCmdScope/3  "HdgCmd"
  Vt/1 -> k2/1
  k2/1 -> Saturation/1  "VTfps"
  k/1 -> Saturation Dynamic1/3
  RollLimit/1 -> k3/1
  Sum3/1 -> Saturation Dynamic1/2  "eaccel"
  Saturation Dynamic1/1 -> VarLimIntegIC/3(In), HdgCmdScope/1  "LimAccel"
  k3/1 -> Trigonometric Function/1
  Trigonometric Function/1 -> k4/1
  k4/1 -> k5/1
  k5/1 -> Product3/1
  Product3/1 -> VarLimIntegIC/1(UpLim), k1/1  "RateLim"
  k1/1 -> VarLimIntegIC/2(LoLim)
  VarLimIntegIC/1(Out) -> Integrator1/1, HdgCmdScope/2, Unit Delay1/1, HdgRteCmd/1  "LimRate"
  k6/1 -> 2zetaOmega/2
  2zetaOmega/1 -> Sum3/2
  init/1 -> VarLimIntegIC/5(IC)
  omegaSq/1 -> omegaSq2/1
  omegaSq2/1 -> Sum3/1
  Sum2/1 -> ANGL/1(in)  "epos"
  HdgCmdMCP/1 -> Logical Operator/1, Sum2/1, HdgCmdScope/4  "Cmd"
  ANGL/1(180) -> omegaSq2/2
  Logical Operator/1 -> VarLimIntegIC/4(Trig), Integrator1/2
  Saturation/1 -> Product1/2, Product2/2, Product3/2
  Heading/1 -> Integrator1/3
  Product2/1 -> Saturation Dynamic1/1, k/1
  Constant/1 -> Sum/1
  Constant1/1 -> Product1/1
  Product1/1 -> Sum/2
  Constant2/1 -> Product2/1
  Sum/1 -> k6/1, omegaSq/1, omegaSq/2  "omega"
  Unit Delay/1 -> Sum2/2
  Unit Delay1/1 -> 2zetaOmega/1

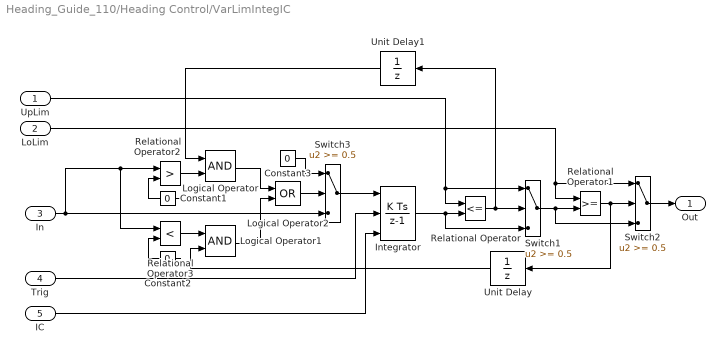
== system Heading_Guide_110/Heading Control/VarLimIntegIC ==
  UpLim : Inport  RequirementInfo={} %GIDa_a52f7b7f_3cd2_4b84_aa46_8f49d190de5c
  LoLim : Inport  RequirementInfo={} %GIDa_14f49477_0466_41ac_a405_ff8b353df89c  Port=2
  In : Inport  RequirementInfo={} %GIDa_3e285f49_2930_4df4_81dd_a9b406bbe3bd  Port=3
  Trig : Inport  RequirementInfo={} %GIDa_a10733bc_08b5_4d2b_a4b2_d21b5a57b6cc  Port=4
  IC : Inport  RequirementInfo={} %GIDa_1f0c5f5f_64dd_4362_ac43_aa1a0320c078  Port=5
  Constant1 : Constant  RequirementInfo={} %GIDa_06ecceb0_a33e_4777_98b5_cbb205f23b1a  Value=0
  Constant2 : Constant  RequirementInfo={} %GIDa_450747a0_c4d7_4d05_b9cd_637cc0a6e70e  Value=0
  Constant3 : Constant  RequirementInfo={} %GIDa_2162f9e8_6490_497e_a11b_22bba3b34cf8  Value=0
  Integrator : DiscreteIntegrator  ExternalReset=level  InitialConditionSource=external  SampleTime=1.0  ICPrevOutput=DiscIntNeverNeededParam  ICPrevScaledInput=DiscIntNeverNeededParam  mask(DiscretizedDiscreteIntegrator){}
      mask init:
      | %zoh
  Logical Operator : Logic  RequirementInfo={} %GIDa_08f35c7f_9ec6_4cc6_9a1f_42b21408c66a  AllPortsSameDT=off
  Logical Operator1 : Logic  RequirementInfo={} %GIDa_78d08ac2_a159_4fb8_990a_70ef898240f1  AllPortsSameDT=off
  Logical Operator2 : Logic  RequirementInfo={} %GIDa_16203443_42bb_4de7_9e01_30a8f399b69b  Operator=OR  AllPortsSameDT=off
  Relational Operator : RelationalOperator  RequirementInfo={} %GIDa_fd2b09f2_7292_41cd_b490_47957a93b770  Operator=<=
  Relational Operator1 : RelationalOperator  RequirementInfo={} %GIDa_bc21e44d_a4ad_4459_a4e5_c40c404b3dbb
  Relational Operator2 : RelationalOperator  RequirementInfo={} %GIDa_257b199b_80e3_40b3_851a_c63ec13dd9de  Operator=>
  Relational Operator3 : RelationalOperator  RequirementInfo={} %GIDa_34126d1c_0a68_4b2a_a8f9_adf647778def  Operator=<
  Switch1 : Switch  RequirementInfo={} %GIDa_093ada51_26d0_4dd4_951b_93ea95402387  Threshold=0.5  SaturateOnIntegerOverflow=on  InputSameDT=on
  Switch2 : Switch  RequirementInfo={} %GIDa_ce0381f3_056e_496f_90b9_8ff8975dbd4b  Threshold=0.5  SaturateOnIntegerOverflow=on  InputSameDT=on
  Switch3 : Switch  RequirementInfo={} %GIDa_23ed59f4_3b4c_47cd_8936_54e05a064030  Threshold=0.5  SaturateOnIntegerOverflow=on  InputSameDT=on
  Unit Delay : UnitDelay  SampleTime=-1
  Unit Delay1 : UnitDelay  SampleTime=-1
  Out : Outport  RequirementInfo={} %GIDa_a2a80f39_47d8_4649_81f4_5246420c0c65
  wires:
  Relational Operator1/1 -> Unit Delay/1, Switch2/2
  Switch1/1 -> Switch2/3, Relational Operator1/2
  LoLim/1 -> Relational Operator1/1, Switch2/1
  IC/1 -> Integrator/3
  Trig/1 -> Integrator/2
  Constant2/1 -> Relational Operator3/2
  Relational Operator3/1 -> Logical Operator1/1
  Logical Operator1/1 -> Logical Operator2/2
  Logical Operator/1 -> Logical Operator2/1
  Logical Operator2/1 -> Switch3/2
  Relational Operator2/1 -> Logical Operator/2
  Constant1/1 -> Relational Operator2/2
  In/1 -> Switch3/3, Relational Operator3/1, Relational Operator2/1
  Constant3/1 -> Switch3/1
  Switch3/1 -> Integrator/1
  Relational Operator/1 -> Unit Delay1/1, Switch1/2
  Switch2/1 -> Out/1
  UpLim/1 -> Switch1/1, Relational Operator/1
  Integrator/1 -> Relational Operator/2, Switch1/3
  Unit Delay/1 -> Logical Operator1/2
  Unit Delay1/1 -> Logical Operator/1

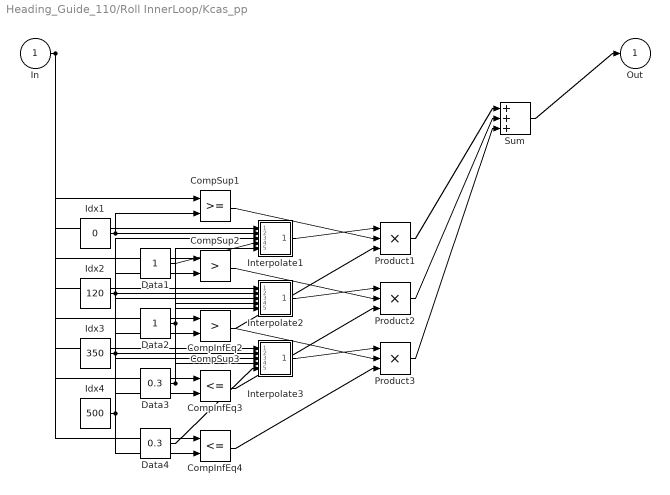
== system Heading_Guide_110/Roll InnerLoop/Kcas_pp ==
  In : Inport
  CompInfEq2 : RelationalOperator  Operator=<=  InputSameDT=on
  CompInfEq3 : RelationalOperator  Operator=<=  InputSameDT=on
  CompInfEq4 : RelationalOperator  Operator=<=  InputSameDT=on
  CompSup1 : RelationalOperator  InputSameDT=on
  CompSup2 : RelationalOperator  Operator=>  InputSameDT=on
  CompSup3 : RelationalOperator  Operator=>  InputSameDT=on
  Data1 : Constant
  Data2 : Constant
  Data3 : Constant  Value=0.3
  Data4 : Constant  Value=0.3
  Idx1 : Constant  Value=0
  Idx2 : Constant  Value=120
  Idx3 : Constant  Value=350
  Idx4 : Constant  Value=500
  Interpolate1 : Subsystem
  Interpolate2 : Subsystem
  Interpolate3 : Subsystem
  Product1 : Product  Inputs=***  SaturateOnIntegerOverflow=on  RndMeth=Zero  OutDataTypeStr=Inherit: Same as first input
  Product2 : Product  Inputs=***  SaturateOnIntegerOverflow=on  RndMeth=Zero  OutDataTypeStr=Inherit: Same as first input
  Product3 : Product  Inputs=***  SaturateOnIntegerOverflow=on  RndMeth=Zero  OutDataTypeStr=Inherit: Same as first input
  Sum : Sum  Inputs=+++  SaturateOnIntegerOverflow=on  InputSameDT=on  OutDataTypeStr=Inherit: Same as first input
  Out : Outport
  wires:
  In/1 -> Interpolate1/1(InportIn), CompSup1/1, Interpolate2/1(InportIn), CompSup2/1, CompInfEq2/1, Interpolate3/1(InportIn), CompSup3/1, CompInfEq3/1, CompInfEq4/1
  Idx1/1 -> Interpolate1/2(InportIdx1), CompSup1/2
  Data1/1 -> Interpolate1/4(InportData1)
  Interpolate1/1(Out) -> Product1/1
  CompSup1/1 -> Product1/2
  CompInfEq2/1 -> Product1/3
  Product1/1 -> Sum/1
  Idx2/1 -> Interpolate2/2(InportIdx1), CompSup2/2, Interpolate1/3(InportIdx2), CompInfEq2/2
  Data2/1 -> Interpolate2/4(InportData1), Interpolate1/5(InportData2)
  Interpolate2/1(Out) -> Product2/1
  CompSup2/1 -> Product2/2
  CompInfEq3/1 -> Product2/3
  Product2/1 -> Sum/2
  Idx3/1 -> Interpolate3/2(InportIdx1), CompSup3/2, Interpolate2/3(InportIdx2), CompInfEq3/2
  Data3/1 -> Interpolate3/4(InportData1), Interpolate2/5(InportData2)
  Interpolate3/1(Out) -> Product3/1
  CompSup3/1 -> Product3/2
  CompInfEq4/1 -> Product3/3
  Product3/1 -> Sum/3
  Idx4/1 -> Interpolate3/3(InportIdx2), CompInfEq4/2
  Data4/1 -> Interpolate3/5(InportData2)
  Sum/1 -> Out/1

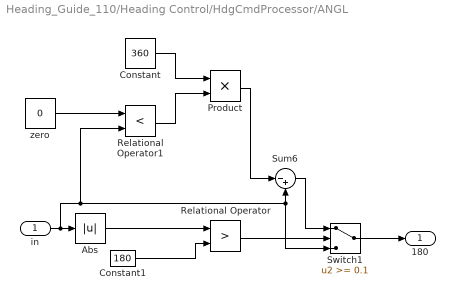
== system Heading_Guide_110/Heading Control/HdgCmdProcessor/ANGL ==
  in : Inport  RequirementInfo={} %GIDa_91f853c7_c908_401d_adfc_518d7751528f
  Abs : Abs
  Constant : Constant  Value=360
  Constant1 : Constant  RequirementInfo={} %GIDa_7c5c3c02_b72b_4cab_88d9_ce8964dea6e5  Value=180
  Product : Product  RndMeth=Zero
  Relational Operator : RelationalOperator  RequirementInfo={} %GIDa_7fca63f4_30c3_4611_a13c_f242258541ac  Operator=>
  Relational Operator1 : RelationalOperator  Operator=<  OutDataTypeStr=boolean
  Sum6 : Sum  RequirementInfo={} %GIDa_8f691f86_6b2c_4343_a08d_01121fff99a8  Inputs=|-+  SaturateOnIntegerOverflow=on
  Switch1 : Switch  RequirementInfo={} %GIDa_9f6a3e17_ac1f_4a7c_b770_43e31d539b0d  Threshold=0.1  SaturateOnIntegerOverflow=on
  zero : Constant  Value=0
  180 : Outport  RequirementInfo={} %GIDa_da671ccf_1469_4f90_9911_e50416dafc2f
  wires:
  Abs/1 -> Relational Operator/1
  in/1 -> Abs/1, Switch1/3, Sum6/2, Relational Operator1/2
  Switch1/1 -> 180/1
  Product/1 -> Sum6/1
  Sum6/1 -> Switch1/1
  Relational Operator/1 -> Switch1/2
  Constant1/1 -> Relational Operator/2
  zero/1 -> Relational Operator1/1
  Constant/1 -> Product/1
  Relational Operator1/1 -> Product/2

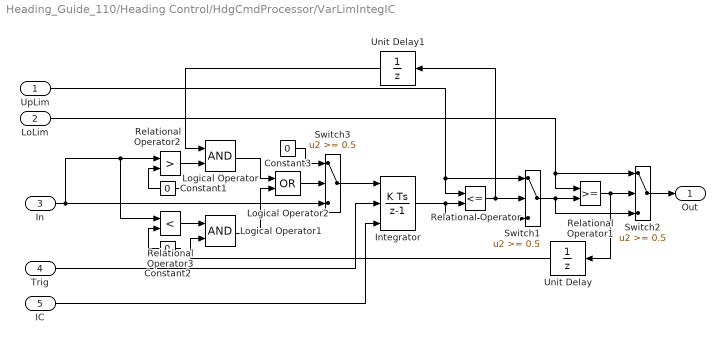
== system Heading_Guide_110/Heading Control/HdgCmdProcessor/VarLimIntegIC ==
  UpLim : Inport  RequirementInfo={} %GIDa_b6974814_32b4_446c_a7b5_2b64616822d2
  LoLim : Inport  RequirementInfo={} %GIDa_b4069f0f_04d2_435d_9d74_47f31e226abc  Port=2
  In : Inport  RequirementInfo={} %GIDa_ffe63698_9663_4b08_a6c4_0cfcc14ab018  Port=3
  Trig : Inport  RequirementInfo={} %GIDa_6297cb9d_5b31_4d8e_a321_41fbf142c5b4  Port=4
  IC : Inport  RequirementInfo={} %GIDa_59f2d505_3cc2_4942_9dd8_a5a4ff923eba  Port=5
  Constant1 : Constant  RequirementInfo={} %GIDa_5f63bf18_9b52_4c75_b33f_d083ba316d1e  Value=0
  Constant2 : Constant  RequirementInfo={} %GIDa_3ef1a0c3_325a_4a1e_87f1_8a7ceb7f2ed7  Value=0
  Constant3 : Constant  RequirementInfo={} %GIDa_3c010cc6_e66d_42da_9a5a_231ebe5e9c3f  Value=0
  Integrator : DiscreteIntegrator  ExternalReset=level  InitialConditionSource=external  SampleTime=1.0  ICPrevOutput=DiscIntNeverNeededParam  ICPrevScaledInput=DiscIntNeverNeededParam  mask(DiscretizedDiscreteIntegrator){}
      mask init:
      | %zoh
  Logical Operator : Logic  RequirementInfo={} %GIDa_a60b4d2f_6552_4cb5_b522_727de66498b0  AllPortsSameDT=off
  Logical Operator1 : Logic  RequirementInfo={} %GIDa_8f81d6cf_a2aa_4e00_869d_ceffbd7871c1  AllPortsSameDT=off
  Logical Operator2 : Logic  RequirementInfo={} %GIDa_6338745d_e0be_46bf_a46f_644f808dad4e  Operator=OR  AllPortsSameDT=off
  Relational Operator : RelationalOperator  RequirementInfo={} %GIDa_8e878cd0_b3b2_4162_9fe2_c686049f0806  Operator=<=
  Relational Operator1 : RelationalOperator  RequirementInfo={} %GIDa_b45a0ded_1a8c_4a6d_a67f_e5d263373459
  Relational Operator2 : RelationalOperator  RequirementInfo={} %GIDa_a0755ed8_a69f_4262_8ce5_c41fc56502ff  Operator=>
  Relational Operator3 : RelationalOperator  RequirementInfo={} %GIDa_8264758e_f6c1_4924_85b8_a6eda5126d21  Operator=<
  Switch1 : Switch  RequirementInfo={} %GIDa_4c3fce01_41f9_40b1_a6a3_6d04c9eccd5a  Threshold=0.5  SaturateOnIntegerOverflow=on  InputSameDT=on
  Switch2 : Switch  RequirementInfo={} %GIDa_b2e7bf7c_7029_45e6_9cda_915a12f41445  Threshold=0.5  SaturateOnIntegerOverflow=on  InputSameDT=on
  Switch3 : Switch  RequirementInfo={} %GIDa_bec6d583_cd7d_4a0e_9481_7e8d505e2b66  Threshold=0.5  SaturateOnIntegerOverflow=on  InputSameDT=on
  Unit Delay : UnitDelay  SampleTime=-1
  Unit Delay1 : UnitDelay  SampleTime=-1
  Out : Outport  RequirementInfo={} %GIDa_6b54eae4_0c2d_43e8_87f0_b15564168c0d
  wires:
  Relational Operator1/1 -> Unit Delay/1, Switch2/2
  Switch1/1 -> Switch2/3, Relational Operator1/2
  LoLim/1 -> Relational Operator1/1, Switch2/1
  IC/1 -> Integrator/3
  Trig/1 -> Integrator/2
  Constant2/1 -> Relational Operator3/2
  Relational Operator3/1 -> Logical Operator1/1
  Logical Operator1/1 -> Logical Operator2/2
  Logical Operator/1 -> Logical Operator2/1
  Logical Operator2/1 -> Switch3/2
  Relational Operator2/1 -> Logical Operator/2
  Constant1/1 -> Relational Operator2/2
  In/1 -> Switch3/3, Relational Operator3/1, Relational Operator2/1
  Constant3/1 -> Switch3/1
  Switch3/1 -> Integrator/1
  Relational Operator/1 -> Unit Delay1/1, Switch1/2
  Switch2/1 -> Out/1
  UpLim/1 -> Switch1/1, Relational Operator/1
  Integrator/1 -> Relational Operator/2, Switch1/3
  Unit Delay/1 -> Logical Operator1/2
  Unit Delay1/1 -> Logical Operator/1

== system Heading_Guide_110/Roll InnerLoop/Kcas_pp/Interpolate1 ==
  InportIn : Inport
  InportIdx1 : Inport  Port=2
  InportIdx2 : Inport  Port=3
  InportData1 : Inport  Port=4
  InportData2 : Inport  Port=5
  Interpolate : Product  Inputs=*/*  SaturateOnIntegerOverflow=on  RndMeth=Zero  InputSameDT=on  OutDataTypeStr=Inherit: Same as first input
  Sum1 : Sum  Inputs=+-  SaturateOnIntegerOverflow=on  InputSameDT=on  OutDataTypeStr=Inherit: Same as first input
  Sum2 : Sum  Inputs=-+  SaturateOnIntegerOverflow=on  InputSameDT=on  OutDataTypeStr=Inherit: Same as first input
  Sum3 : Sum  Inputs=-+  SaturateOnIntegerOverflow=on  InputSameDT=on  OutDataTypeStr=Inherit: Same as first input
  Sum4 : Sum  SaturateOnIntegerOverflow=on  InputSameDT=on  OutDataTypeStr=Inherit: Same as first input
  Out : Outport
  wires:
  InportIn/1 -> Sum1/1
  InportIdx1/1 -> Sum1/2, Sum2/1
  InportIdx2/1 -> Sum2/2
  InportData1/1 -> Sum3/1, Sum4/2
  InportData2/1 -> Sum3/2
  Sum1/1 -> Interpolate/1
  Sum2/1 -> Interpolate/2
  Sum3/1 -> Interpolate/3
  Interpolate/1 -> Sum4/1
  Sum4/1 -> Out/1

== system Heading_Guide_110/Roll InnerLoop/Kcas_pp/Interpolate2 ==
  InportIn : Inport
  InportIdx1 : Inport  Port=2
  InportIdx2 : Inport  Port=3
  InportData1 : Inport  Port=4
  InportData2 : Inport  Port=5
  Interpolate : Product  Inputs=*/*  SaturateOnIntegerOverflow=on  RndMeth=Zero  InputSameDT=on  OutDataTypeStr=Inherit: Same as first input
  Sum1 : Sum  Inputs=+-  SaturateOnIntegerOverflow=on  InputSameDT=on  OutDataTypeStr=Inherit: Same as first input
  Sum2 : Sum  Inputs=-+  SaturateOnIntegerOverflow=on  InputSameDT=on  OutDataTypeStr=Inherit: Same as first input
  Sum3 : Sum  Inputs=-+  SaturateOnIntegerOverflow=on  InputSameDT=on  OutDataTypeStr=Inherit: Same as first input
  Sum4 : Sum  SaturateOnIntegerOverflow=on  InputSameDT=on  OutDataTypeStr=Inherit: Same as first input
  Out : Outport
  wires:
  InportIn/1 -> Sum1/1
  InportIdx1/1 -> Sum1/2, Sum2/1
  InportIdx2/1 -> Sum2/2
  InportData1/1 -> Sum3/1, Sum4/2
  InportData2/1 -> Sum3/2
  Sum1/1 -> Interpolate/1
  Sum2/1 -> Interpolate/2
  Sum3/1 -> Interpolate/3
  Interpolate/1 -> Sum4/1
  Sum4/1 -> Out/1

== system Heading_Guide_110/Roll InnerLoop/Kcas_pp/Interpolate3 ==
  InportIn : Inport
  InportIdx1 : Inport  Port=2
  InportIdx2 : Inport  Port=3
  InportData1 : Inport  Port=4
  InportData2 : Inport  Port=5
  Interpolate : Product  Inputs=*/*  SaturateOnIntegerOverflow=on  RndMeth=Zero  InputSameDT=on  OutDataTypeStr=Inherit: Same as first input
  Sum1 : Sum  Inputs=+-  SaturateOnIntegerOverflow=on  InputSameDT=on  OutDataTypeStr=Inherit: Same as first input
  Sum2 : Sum  Inputs=-+  SaturateOnIntegerOverflow=on  InputSameDT=on  OutDataTypeStr=Inherit: Same as first input
  Sum3 : Sum  Inputs=-+  SaturateOnIntegerOverflow=on  InputSameDT=on  OutDataTypeStr=Inherit: Same as first input
  Sum4 : Sum  SaturateOnIntegerOverflow=on  InputSameDT=on  OutDataTypeStr=Inherit: Same as first input
  Out : Outport
  wires:
  InportIn/1 -> Sum1/1
  InportIdx1/1 -> Sum1/2, Sum2/1
  InportIdx2/1 -> Sum2/2
  InportData1/1 -> Sum3/1, Sum4/2
  InportData2/1 -> Sum3/2
  Sum1/1 -> Interpolate/1
  Sum2/1 -> Interpolate/2
  Sum3/1 -> Interpolate/3
  Interpolate/1 -> Sum4/1
  Sum4/1 -> Out/1
